simulink model "RLvali_2021bold"  (R2021b)
settings: Solver=ode15s  StartTime=0.0  StopTime=Tf  FixedStep=0.01  MaxStep=0.05  RelTol=0.5  AbsTol=0.5
model workspace (MATLAB code in the model file):
  | %---------------Critical values---------------%
  | angle_amp = pi/6; % Motor rotate amplitude, ref: pi/4
  | rotateCorrectionCoef = 1.158;
  | criticalFn = 2;
  | 
  | %------values for normalization---------------%
  | % values got by running manual gait
  | rotxNormGain = 1/0.1;
  | rotyNormGain = 1/0.05;
  | rotzNormGain = 1/0.1;
  | 
  | vxNormGain = 1/0.2;
  | vyNormGain = 1/0.2;
  | vzNormGain = 1/0.2;
  | 
  | FnNormGain = 1/15;
  | 
  | %--------values for check done---------------%
  | rotDone = pi/6; % 0.15;
  | legBendDone = pi/3; % actuator max bending angle
  | 
  | 
  | %---------------Robot parameters-------------%
  | % robot size
  | robot_width = 0.15;
  | robot_length = 0.22;
  | 
  | % floor parameters
  | floor_length = 2;
  | floor_width = 2;
  | 
  | % continuum actuator size
  | L_disk = 0.02944;% Disk side length (m)
  | R_w = L_disk/sqrt(3);
  | thickness_disk = 0.004; % Disk thickness (m)
  | thigh_length = 0.06;
  | R_core = 0.005; % Core radius (m)
  | length_core = 0.008; % Core length (m)
  | R_spool = 0.021; % 0.01944; % radius of the spool
  | spool_height = 0.022+0.015;
  | R_pulley = 1e-3;
  | spool_k = 0;
  | spool_d = 0;
  | hole_d = 4e-3;
  | 
  | % Material property
  | rho_PLA = 1.24e3;
  | rho = 1.19e3; % 1.19e3; % Density (kg/m^3)
  | % use rigid joints
  | Pz_stiff = 135000;
  | Pz_damping = 500;
  | S_stiff = 0.0239;
  | S_damping = 7.5e-5;
  | S_low_Bound = -20;
  | S_up_Bound = 20;
  | 
  | R_foot = 0.015; % foot radius (m)
  | 
  | % motor parameter
  | stall_T = 11.2/10; % 11.2 cm*kg, stall torque
  | t_60_deg = 0.2; % 0.09 s
  | V_nomrmal = 6; % corresponding normal voltage
  | Jr = 0.0001; %g*cm^2, robot inertia
  | 
  | % contact force
  | coef_static_friction = 0.315;
  | coef_dynamic_friction = 0.3;
  | crictic_velocity = 0.3; % m/s
  | contact_suf_stiff = 1000; % N/m
  | contact_suf_damp = 50; % N/(m/s)
  | contact_region_width = 2e-3; % m
  | spoolOpacity = 0;
  | tendonColor = [0.902 0.902 0.902];
  | tendonOpacity = 0.1;
  | 
  | % If use point masses
  | MMainFrame = 198; % g
  | MServoMotor = 50.55;
  | MMotorSupport = 12.1;
  | MSpool = 9.2;
  | 
  | % Robot total weight about 2 kg
  | MComposateLoad = 200;
  | 
  | MBuck = 40; % x2
  | MPCB_RPi = 141.3;
  | MLiBattery = 120; % x2
  | MPowerBank = 66.5;
  | isLoadVisible = 0.1;
  | 
  | 
  | MThigh = 26.7963;
  | MCore = 0.747699;
  | MDisk = 1.78642;
  | MFoot = 16.8232;
values from neighbouring files (symbols this model uses):
  N = ceil((A - 8) / (2.285 * abs(Wstop(1) - Wpass(1))))    [testit.m]
  Tf = 10    [longTest.m]    (also in singleTest.m)
  Ts = 0.05    [longTest.m]    (also in singleTest.m)
  x_norm_min = min(x,[],1)    [preprocessData.m]
  x_norm_range = max(x,[],1) - min(x,[],1)    [preprocessData.m]
  y_norm_min = min(y,[],1)    [preprocessData.m]
  y_norm_range = max(y,[],1) - min(y,[],1)    [preprocessData.m]
undefined symbols (not defined in the file or in its folder): alpha_b_gain, alpha_r_gain, DCMotor_K, EntropyList, EntropyWeightList, ExtParts, fnVariance, isCheckDone, isContactBoolean, isUseExtAct, MotorSupport, rotVariance, speedVariance, startAgentTime, TrackStarServo, VRef, WheelCAD, X, Y, Z, z_l_gain
libraries: sm_lib x311, nesl_utility x81, fl_lib x60, ee_lib x24, simulink x16, slpidlib x12, dspstat3 x2, rllib x1
(part 1 of 16)
settings Model: Creator=Qinglei Ji  LastModifiedBy=4DLab5
settings SolverCC: AutoScaleAbsTol=off  MaxConsecutiveZCs=100  MaxConsecutiveMinStep=10  DaesscMode=Fast  AutoInsertRateTranBlk=on
settings ExplorerConfigSet: InternalSimMechanicsExplorerSettings="<ExplorerConfiguration><canonicalview>default</canonicalview><AnimationSetting><BasePlaybackSpeed>1.0</BasePlaybackSpeed><PlaybackSpeedFactor>1.0</PlaybackSpeedFactor></AnimationSetting><TilePanel><TileInfo><Tiles Columns=\"1\" Count=\"1\" Rows=\"1\"><Column Weight=\"1\"/><Row Weight=\"1\"/><Tile Height=\"1\" Width=\"1\" X=\"0\" Y=\"0\"/></Tiles></TileInfo><SceneInfo><SceneViewer><BGColor><R>0.60000002384185791</R><G>0.60000002384185791</G><B>0.60000002384185791</B></BGColor><Camera><DoPerspective>off</DoPerspective><Position><X>-18.8331461547739707</X><Y>25.880517186070815</Y><Z>26.8100820833696147</Z></Position><Center><X>0.29785977478998571</X><Y>-0.293010908258582892</Y><Z>-0.346783787749327221</Z></Center><Up><X>0.517886432622382209</X><Y>-0.40389178028612327</Y><Z>0.754098848111419029</Z></Up><ViewLimDist>1</ViewLimDist><YLim>0.421333194645766129</YLim><XLim>0.456755011894746488</XLim></Camera></SceneViewer></SceneInfo></TilePanel><MechEditorPanel><Cameras/><GfxPanelCameraMap/><VideoCreator><PlaybackSpeedRatio>1.0</PlaybackSpeedRatio><FrameRate>60</FrameRate><VideoFormat>MPEG-4</VideoFormat><FrameSize>auto</FrameSize></VideoCreator></MechEditorPanel></ExplorerConfiguration>"

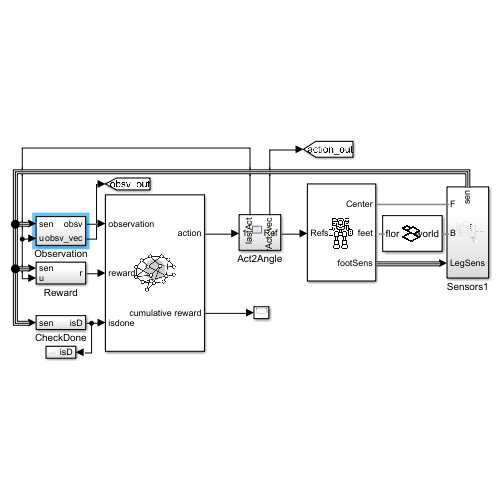
[thumbnail: Simulink's stored preview of the top-level diagram]
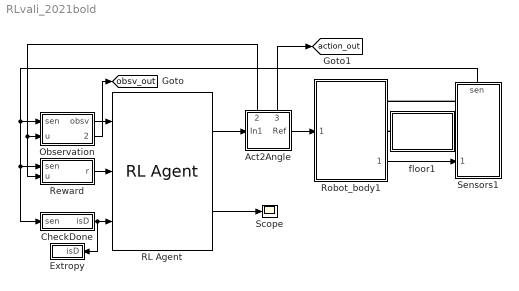
== system RLvali_2021bold ==
  Act2Angle : Subsystem
      settings: PortSchema="{\"entries\":[{\"content\":{\"sides\":[{\"content\":{\"connectorIds\":[\"In1\"]},\"type\":\"ConnectorPlacement.EquallySpacedRectSide\",\"uuid\":\"f23e08d3-9737-483d-bbfd-3ecb6f48fb39\"},{\"content\":{\"connectorIds\":[\"Out1\"],\"side\":\"RIGHT\"},\"type\":\"ConnectorPlacement.EquallySpacedRectSide\",\"uuid\":\"8d685ed7-5054-4615-a3e0-c1ab4f56a55e\"},{\"content\":{\"connectorIds\":[\"Out2\",\"Out3\"],\"side\":\"TOP\"},\"type\":\"ConnectorPlacement.EquallySpacedRectSide\",\"uuid\":\"34bb8f53-1c44-464f-ad5f-1618b85759f2\"}]},\"type\":\"ConnectorPlacement.EquallySpacedConnector\",\"uuid\":\"6728473f-c42e-49f1-b1f4-018a95208548\"}],\"packageUris\":[\"http://schema.mathworks.com/mf0/Connector/R2020b\"],\"version\":\"1.0\"}"
  CheckDone : Subsystem
  Extropy : Subsystem
  Observation : Subsystem
  RL Agent : rllib/RL Agent  Agent=agent  ExternalActionAsInput=off  ProvideCumRwd=on  TreatAsDirectFeedthrough=on
  Reward : Subsystem
  Robot_body1 : Subsystem
      settings: PortSchema="{\"entries\":[{\"content\":{\"sides\":[{\"content\":{\"connectorIds\":[]},\"type\":\"ConnectorPlacement.EquallySpacedRectSide\",\"uuid\":\"6da386a3-61dc-48ac-8951-5f405dad6f0b\"},{\"content\":{\"connectorIds\":[],\"side\":\"RIGHT\"},\"type\":\"ConnectorPlacement.EquallySpacedRectSide\",\"uuid\":\"f31d08fd-e336-4992-a7a1-a5f80310301f\"},{\"content\":{\"connectorIds\":[\"In1\"],\"side\":\"TOP\"},\"type\":\"ConnectorPlacement.EquallySpacedRectSide\",\"uuid\":\"e8d57c74-e878-4fd7-b952-570b3b82c07d\"},{\"content\":{\"connectorIds\":[\"RConn1\",\"RConn2\",\"Out1\"],\"side\":\"BOTTOM\"},\"type\":\"ConnectorPlacement.EquallySpacedRectSide\",\"uuid\":\"5cd044ae-e3eb-4740-b1cb-bb65851cb112\"}]},\"type\":\"ConnectorPlacement.EquallySpacedConnector\",\"uuid\":\"f9915cad-378a-4c2b-ad9c-362eed90ff8c\"}],\"packageUris\":[\"http://schema.mathworks.com/mf0/Connector/R2020b\"],\"version\":\"1.0\"}"
      mask Display: image('$imagefile'); % Use "Edit Image" on toolstrip to change.
  Scope : Scope
  Sensors1 : Subsystem
      settings: PortSchema="{\"entries\":[{\"content\":{\"sides\":[{\"content\":{\"connectorIds\":[\"LConn1\",\"LConn2\",\"In1\"]},\"type\":\"ConnectorPlacement.EquallySpacedRectSide\",\"uuid\":\"4b5ddd47-03f4-426a-88ee-d6acf531c637\"},{\"content\":{\"connectorIds\":[],\"side\":\"RIGHT\"},\"type\":\"ConnectorPlacement.EquallySpacedRectSide\",\"uuid\":\"f2192e31-fae6-4bce-a663-c668a18a2c9c\"},{\"content\":{\"connectorIds\":[\"Out1\"],\"side\":\"TOP\"},\"type\":\"ConnectorPlacement.EquallySpacedRectSide\",\"uuid\":\"20a91eaf-2ad2-4a0d-933a-434c603de7e7\"},{\"content\":{\"connectorIds\":[],\"side\":\"BOTTOM\"},\"type\":\"ConnectorPlacement.EquallySpacedRectSide\",\"uuid\":\"f2757d81-d7c7-43da-8561-08295a517c19\"}]},\"type\":\"ConnectorPlacement.EquallySpacedConnector\",\"uuid\":\"8ce371b8-5669-40c8-963e-855906aef91d\"}],\"packageUris\":[\"http://schema.mathworks.com/mf0/Connector/R2020b\"],\"version\":\"1.0\"}"
  floor1 : Subsystem
      mask Display: image('$imagefile'); % Use "Edit Image" on toolstrip to change.
  tag scope: action_out=global, obsv_out=global
  wires:
  Reward/1(r) -> RL Agent/2
  RL Agent/2 -> Scope/1
  Sensors1/1(sen) -> CheckDone/1(sen), Reward/1(sen), Observation/1(sen)
  CheckDone/1(isD) -> Extropy/1(isD), RL Agent/3
  Observation/1(obsv) -> RL Agent/1
  Act2Angle/1(Ref) -> Robot_body1/1(motorRefs)
  RL Agent/1 -> Act2Angle/1(In1)
  Observation/2(obsv_vec) -> [obsv_out]
  Act2Angle/3(currAct_vec) -> [action_out]
  Act2Angle/2(lastAct) -> Reward/2(u), Observation/2(u)
  Robot_body1/1(footSens) -> Sensors1/1(LegSens)
  connections:
  Sensors1/LConn1 -- Robot_body1/RConn1
  floor1/RConn1 -- Robot_body1/RConn2
  floor1/LConn1 -- Sensors1/LConn2

== system RLvali_2021bold/Act2Angle ==
  note: Learn motor ref
  In1 : Inport
  DecideToUseExt : Subsystem
  Delay : Delay  DelayLength=1  InitialCondition=[0.5;0.5;0.5;0.5]
  Human expert : Subsystem  Commented=on
  Human expert1 : Subsystem
  Subsystem1 : Subsystem  Commented=on
  Subsystem2 : Subsystem
  action2angle : Subsystem  Commented=on
  useExt? : Switch  Criteria=u2 > Threshold
  Ref : Outport
  lastAct : Outport  Port=2
  currAct_vec : Outport  Port=3
  wires:
  In1/1 -> useExt?/3  "Acts"
  Subsystem2/1(refs) -> Ref/1
  Delay/1 -> lastAct/1
  useExt?/1 -> Subsystem2/1(Acts), Delay/1, currAct_vec/1
  DecideToUseExt/1(Out1) -> useExt?/2
  Human expert1/1(Inport) -> useExt?/1

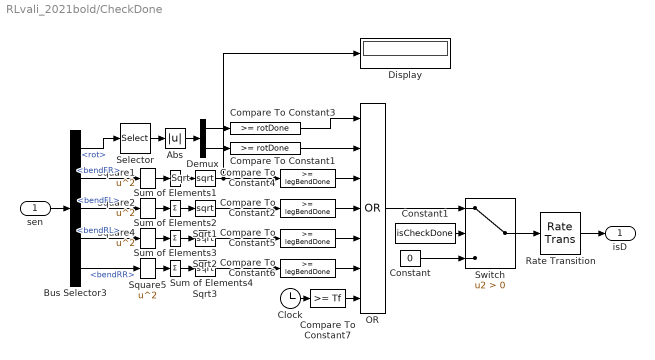
== system RLvali_2021bold/CheckDone ==
  sen : Inport
  Abs : Abs
  Bus Selector3 : BusSelector  OutputSignals=rot,SigsFromLegs.bendFR,SigsFromLegs.bendFL,SigsFromLegs.bendRL,SigsFromLegs.bendRR
  Clock : Clock
  Compare To Constant1 : simulink/Logic and Bit Operations/Compare To Constant  relop=>=  const=rotDone  OutDataTypeStr=boolean
  Compare To Constant{2,4..6} (4 alike) : simulink/Logic and Bit Operations/Compare To Constant  relop=>=  const=legBendDone  OutDataTypeStr=boolean
  Compare To Constant3 : simulink/Logic and Bit Operations/Compare To Constant  relop=>=  const=rotDone  OutDataTypeStr=boolean
  Compare To Constant7 : simulink/Logic and Bit Operations/Compare To Constant  relop=>=  const=Tf  OutDataTypeStr=boolean
  Constant : Constant  Value=0
  Constant1 : Constant  Value=isCheckDone
  Demux : Demux  Outputs=2
  Display : Display
  OR : Logic  Operator=OR  Inputs=7  AllPortsSameDT=off  OutDataTypeStr=boolean
  Rate Transition : RateTransition
  Selector : Selector  InputPortWidth=3  IndexOptions=Index vector (dialog)  Indices=[1 2]  OutputSizes=1
  Sqrt{,1..3} (4 alike) : Sqrt  SaturateOnIntegerOverflow=on
  Square{1..2,4..5} (4 alike) : Math  Operator=square  SignedPower=on  SaturateOnIntegerOverflow=on
  Sum of Elements{1..4} (4 alike) : Sum  Inputs=+
  Switch : Switch  Criteria=u2 > Threshold
  isD : Outport  VectorParamsAs1DForOutWhenUnconnected=off
  wires:
  Rate Transition/1 -> isD/1
  sen/1 -> Bus Selector3/1
  Bus Selector3/1 -> Selector/1  "<rot>"
  Compare To Constant3/1 -> OR/1
  Bus Selector3/2 -> Square1/1  "<bendFR>"
  Compare To Constant4/1 -> OR/3
  Square1/1 -> Sum of Elements1/1
  Sum of Elements1/1 -> Sqrt/1
  Sqrt/1 -> Compare To Constant4/1, Display/1
  Square2/1 -> Sum of Elements2/1
  Sqrt1/1 -> Compare To Constant2/1
  Sum of Elements2/1 -> Sqrt1/1
  Bus Selector3/3 -> Square2/1  "<bendFL>"
  Compare To Constant2/1 -> OR/4
  Square4/1 -> Sum of Elements3/1
  Sqrt2/1 -> Compare To Constant5/1
  Sum of Elements3/1 -> Sqrt2/1
  Bus Selector3/4 -> Square4/1  "<bendRL>"
  Compare To Constant5/1 -> OR/5
  Square5/1 -> Sum of Elements4/1
  Sqrt3/1 -> Compare To Constant6/1
  Sum of Elements4/1 -> Sqrt3/1
  Bus Selector3/5 -> Square5/1  "<bendRR>"
  Compare To Constant6/1 -> OR/6
  OR/1 -> Switch/1
  Switch/1 -> Rate Transition/1
  Constant/1 -> Switch/3
  Constant1/1 -> Switch/2
  Demux/1 -> Compare To Constant3/1
  Demux/2 -> Compare To Constant1/1
  Compare To Constant1/1 -> OR/2
  Clock/1 -> Compare To Constant7/1
  Compare To Constant7/1 -> OR/7
  Abs/1 -> Demux/1
  Selector/1 -> Abs/1

== system RLvali_2021bold/Extropy ==
  isD : Inport
  Clock : Clock
  Constant : Constant  Value=EntropyWeightList  SampleTime=Ts
  Constant2 : Constant  Value=EntropyList  SampleTime=Ts
  Display : Display
  MATLAB Function : MATLAB Function  TreatAsAtomicUnit=on  SystemSampleTime=Ts
  MATLAB Function1 : MATLAB Function  TreatAsAtomicUnit=on
  wires:
  Constant2/1 -> MATLAB Function/2(EntropyList)  "entropy"
  Constant/1 -> MATLAB Function/1(EntropyWeightList)  "entroWeight"
  isD/1 -> Display/1, MATLAB Function/3(isDone)
  [obsv_out] -> MATLAB Function1/2(obsv)
  [action_out] -> MATLAB Function1/3(act)
  Clock/1 -> MATLAB Function1/1(time)

== system RLvali_2021bold/Observation ==
  sen : Inport
  u : Inport  Port=2
  Mux : Mux
  Mux1 : Mux  Inputs=3
  Mux2 : Mux  Inputs=3
  Mux4 : Mux
  Rate Transition : RateTransition  OutPortSampleTime=Ts
  Subsystem : Subsystem
  contactConversion : Subsystem
  contactConversion1 : Subsystem
  contactConversion2 : Subsystem
  contactConversion3 : Subsystem
  correct : Subsystem  Commented=on
  rotNoise : Subsystem
  rotNoise1 : Subsystem
  rotNoise2 : Subsystem
  speednoise : Subsystem
  speednoise1 : Subsystem
  speednoise2 : Subsystem
  obsv : Outport  VectorParamsAs1DForOutWhenUnconnected=off
  obsv_vec : Outport  Port=2  VectorParamsAs1DForOutWhenUnconnected=off
  wires:
  Mux/1 -> Rate Transition/1
  Rate Transition/1 -> obsv/1
  u/1 -> Mux/4
  Mux1/1 -> Mux/1
  Mux2/1 -> Mux/2
  contactConversion/1(FnOut) -> Mux4/1
  contactConversion1/1(FnOut) -> Mux4/2
  contactConversion2/1(FnOut) -> Mux4/3
  contactConversion3/1(FnOut) -> Mux4/4
  Mux4/1 -> Mux/3
  speednoise/1(Out1) -> Mux2/1
  speednoise1/1(Out1) -> Mux2/2
  speednoise2/1(Out1) -> Mux2/3
  rotNoise/1(Out1) -> Mux1/1
  rotNoise1/1(Out1) -> Mux1/2
  rotNoise2/1(Out1) -> Mux1/3
  sen/1 -> Subsystem/1(In1)
  Subsystem/1(obsv_vec) -> obsv_vec/1
  Subsystem/2(norm) -> rotNoise/1(<vx>)
  Subsystem/3(norm1) -> rotNoise1/1(<vx>)
  Subsystem/4(norm2) -> rotNoise2/1(<vx>)
  Subsystem/5(norm3) -> speednoise/1(<vx>)
  Subsystem/6(norm4) -> speednoise1/1(<vx>)
  Subsystem/7(norm5) -> speednoise2/1(<vx>)
  Subsystem/8(norm6) -> contactConversion/1(Fn)
  Subsystem/9(norm7) -> contactConversion1/1(Fn)
  Subsystem/10(norm8) -> contactConversion2/1(Fn)
  Subsystem/11(norm9) -> contactConversion3/1(Fn)

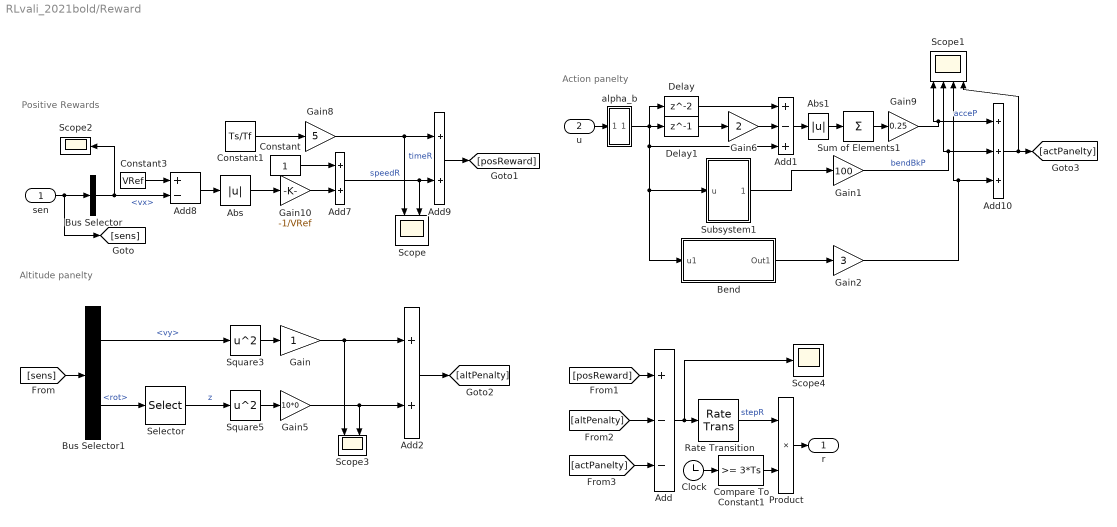
== system RLvali_2021bold/Reward ==
  note: Action panelty
  note: Altitude panelty
  note: Positive Rewards
  sen : Inport
  u : Inport  Port=2
  Abs : Abs
  Abs1 : Abs
  Add : Sum  Inputs=+--
  Add1 : Sum  Inputs=+-+
  Add10 : Sum  Inputs=+++
  Add2 : Sum
  Add7 : Sum
  Add8 : Sum  Inputs=+-
  Add9 : Sum
  Bend : Subsystem
  Bus Selector : BusSelector  OutputSignals=vx
  Bus Selector1 : BusSelector  OutputSignals=vy,rot
  Clock : Clock
  Compare To Constant1 : simulink/Logic and Bit Operations/Compare To Constant  relop=>=  const=3*Ts  OutDataTypeStr=boolean
  Constant : Constant
  Constant1 : Constant  Value=Ts/Tf
  Constant3 : Constant  Value=VRef
  Delay : Delay  InitialCondition=0.5
  Delay1 : Delay  DelayLength=1  InitialCondition=0.5
  Gain : Gain
  Gain1 : Gain  Gain=100
  Gain10 : Gain  Gain=-1/VRef
  Gain2 : Gain  Gain=3
  Gain5 : Gain  Gain=10*0
  Gain6 : Gain  Gain=2
  Gain8 : Gain  Gain=5
  Gain9 : Gain  Gain=0.25
  Product : Product
  Rate Transition : RateTransition  OutPortSampleTime=Ts
  Scope : Scope  NumInputPorts=2
  Scope1 : Scope  NumInputPorts=4
  Scope2 : Scope
  Scope3 : Scope  NumInputPorts=2
  Scope4 : Scope
  Selector : Selector  InputPortWidth=3  IndexOptions=Index vector (dialog)  Indices=[3]  OutputSizes=1
  Square3 : Math  Operator=square  SignedPower=on  SaturateOnIntegerOverflow=on
  Square5 : Math  Operator=square  SignedPower=on  SaturateOnIntegerOverflow=on
  Subsystem1 : Subsystem
  Sum of Elements1 : Sum  Inputs=+
  alpha_b : Subsystem
  r : Outport  VectorParamsAs1DForOutWhenUnconnected=off
  wires:
  sen/1 -> Bus Selector/1, [sens]
  Square3/1 -> Gain/1
  Square5/1 -> Gain5/1
  Selector/1 -> Square5/1  "z"
  Gain/1 -> Scope3/1, Add2/1
  Add/1 -> Scope4/1, Rate Transition/1
  Constant1/1 -> Gain8/1
  Delay/1 -> Add1/1
  Gain6/1 -> Add1/2
  Add1/1 -> Abs1/1
  Abs1/1 -> Sum of Elements1/1
  Delay1/1 -> Gain6/1
  Sum of Elements1/1 -> Gain9/1
  Clock/1 -> Compare To Constant1/1
  Compare To Constant1/1 -> Product/2
  Rate Transition/1 -> Product/1  "stepR"
  Product/1 -> r/1
  [sens] -> Bus Selector1/1
  Gain8/1 -> Add9/1, Scope/1  "timeR"
  Add9/1 -> [posReward]
  Bus Selector1/1 -> Square3/1  "<vy>"
  Bus Selector1/2 -> Selector/1  "<rot>"
  Gain5/1 -> Add2/2, Scope3/2
  Add2/1 -> [altPenalty]
  Gain9/1 -> Add10/1, Scope1/1  "acceP"
  [posReward] -> Add/1
  [altPenalty] -> Add/2
  [actPanelty] -> Add/3
  Add8/1 -> Abs/1
  Constant3/1 -> Add8/1
  Add7/1 -> Scope/2, Add9/2  "speedR"
  Gain10/1 -> Add7/2
  Abs/1 -> Gain10/1
  Constant/1 -> Add7/1
  Subsystem1/1(Out1) -> Gain1/1
  Gain1/1 -> Add10/2, Scope1/2  "bendBkP"
  Add10/1 -> Scope1/4, [actPanelty]
  alpha_b/1(b) -> Bend/1(u1), Subsystem1/1(u), Add1/3, Delay/1, Delay1/1
  u/1 -> alpha_b/1(u)
  Bend/1(Out1) -> Gain2/1
  Gain2/1 -> Scope1/3, Add10/3
  Bus Selector/1 -> Scope2/1, Add8/2  "<vx>"

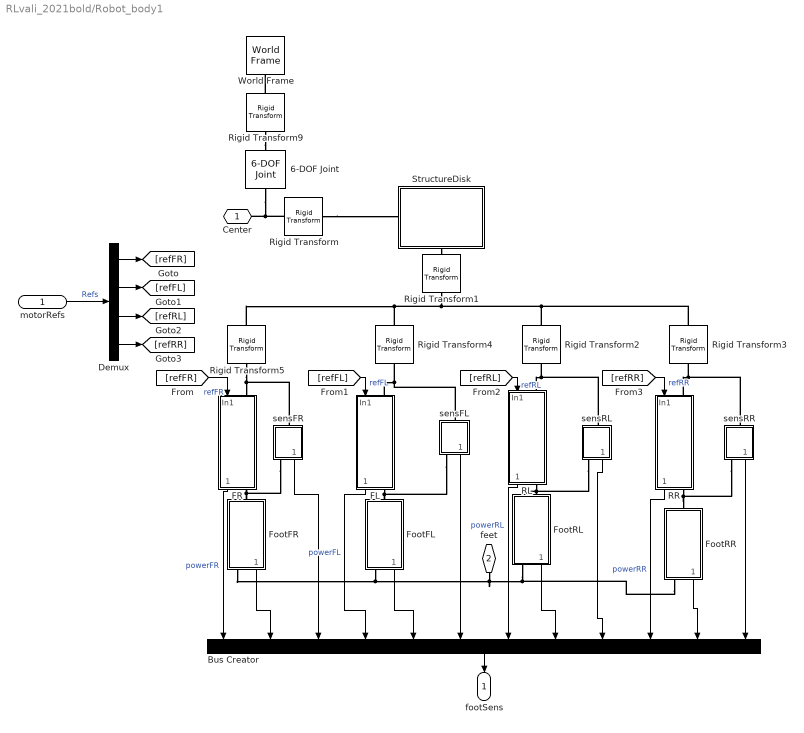
== system RLvali_2021bold/Robot_body1 ==
  motorRefs : Inport
  6-DOF Joint : sm_lib/Joints/6-DOF Joint  JointMode=Normal  SenseConstraintForce=off  SenseConstraintForceX=off  SenseConstraintForceY=off  SenseConstraintForceZ=off  SenseConstraintTorque=off  SenseConstraintTorqueX=off  SenseConstraintTorqueY=off  SenseConstraintTorqueZ=off  SenseTotalForce=off  SenseTotalForceX=off  SenseTotalForceY=off  SenseTotalForceZ=off  SenseTotalTorque=off  SenseTotalTorqueX=off  SenseTotalTorqueY=off  SenseTotalTorqueZ=off  CompositeWrenchDir=FollowerOnBase  CompositeWrenchFrame=BaseFrame  PxEquilibriumPosition=0  PxEquilibriumPositionUnits=m  PxSpringStiffness=0  PxSpringStiffnessUnits=N/m  PxDampingCoefficient=0  PxDampingCoefficientUnits=N/(m/s)  PxTorqueActuationMode=NoTorque  PxMotionActuationMode=ComputedMotion  PxSensePosition=off  PxSenseVelocity=off  PxSenseAcceleration=off  PxSenseTorqueForce=off  PxSenseLowerLimitTorqueForce=off  PxSenseUpperLimitTorqueForce=off  PxLowerLimitSpecify=off  PxLowerLimitBound=-1  PxLowerLimitBoundUnits=m  PxLowerLimitStiffness=1e6  PxLowerLimitStiffnessUnits=N/m  PxLowerLimitDamping=1e3  PxLowerLimitDampingUnits=N/(m/s)  PxLowerLimitTransitionRegionWidth=1e-4  PxLowerLimitTransitionRegionWidthUnits=m  PxUpperLimitSpecify=off  PxUpperLimitBound=1  PxUpperLimitBoundUnits=m  PxUpperLimitStiffness=1e6  PxUpperLimitStiffnessUnits=N/m  PxUpperLimitDamping=1e3  PxUpperLimitDampingUnits=N/(m/s)  PxUpperLimitTransitionRegionWidth=1e-4  PxUpperLimitTransitionRegionWidthUnits=m  PxPositionTargetSpecify=off  PxPositionTargetPriority=High  PxPositionTargetValue=0  PxPositionTargetValueUnits=m  PxVelocityTargetSpecify=off  PxVelocityTargetPriority=High  PxVelocityTargetValue=0  PxVelocityTargetValueUnits=m/s  PyEquilibriumPosition=0  PyEquilibriumPositionUnits=m  PySpringStiffness=0  PySpringStiffnessUnits=N/m  PyDampingCoefficient=0  PyDampingCoefficientUnits=N/(m/s)  PyTorqueActuationMode=NoTorque  PyMotionActuationMode=ComputedMotion  PySensePosition=off  PySenseVelocity=off  PySenseAcceleration=off  PySenseTorqueForce=off  PySenseLowerLimitTorqueForce=off  PySenseUpperLimitTorqueForce=off  PyLowerLimitSpecify=off  PyLowerLimitBound=-1  PyLowerLimitBoundUnits=m  PyLowerLimitStiffness=1e6  PyLowerLimitStiffnessUnits=N/m  PyLowerLimitDamping=1e3  PyLowerLimitDampingUnits=N/(m/s)  PyLowerLimitTransitionRegionWidth=1e-4  PyLowerLimitTransitionRegionWidthUnits=m  PyUpperLimitSpecify=off  PyUpperLimitBound=1  PyUpperLimitBoundUnits=m  PyUpperLimitStiffness=1e6  PyUpperLimitStiffnessUnits=N/m  PyUpperLimitDamping=1e3  PyUpperLimitDampingUnits=N/(m/s)  PyUpperLimitTransitionRegionWidth=1e-4  PyUpperLimitTransitionRegionWidthUnits=m  PyPositionTargetSpecify=off  PyPositionTargetPriority=High  PyPositionTargetValue=0  PyPositionTargetValueUnits=m  PyVelocityTargetSpecify=off  PyVelocityTargetPriority=High  PyVelocityTargetValue=0  PyVelocityTargetValueUnits=m/s  PzEquilibriumPosition=0  PzEquilibriumPositionUnits=m  PzSpringStiffness=0  PzSpringStiffnessUnits=N/m  PzDampingCoefficient=0  PzDampingCoefficientUnits=N/(m/s)  PzTorqueActuationMode=NoTorque  PzMotionActuationMode=ComputedMotion  PzSensePosition=off  PzSenseVelocity=off  PzSenseAcceleration=off  PzSenseTorqueForce=off  PzSenseLowerLimitTorqueForce=off  PzSenseUpperLimitTorqueForce=off  PzLowerLimitSpecify=off  PzLowerLimitBound=-1  PzLowerLimitBoundUnits=m  PzLowerLimitStiffness=1e6  PzLowerLimitStiffnessUnits=N/m  PzLowerLimitDamping=1e3  PzLowerLimitDampingUnits=N/(m/s)  PzLowerLimitTransitionRegionWidth=1e-4  PzLowerLimitTransitionRegionWidthUnits=m  PzUpperLimitSpecify=off  PzUpperLimitBound=1  PzUpperLimitBoundUnits=m  PzUpperLimitStiffness=1e6  PzUpperLimitStiffnessUnits=N/m  PzUpperLimitDamping=1e3  PzUpperLimitDampingUnits=N/(m/s)  PzUpperLimitTransitionRegionWidth=1e-4  PzUpperLimitTransitionRegionWidthUnits=m  PzPositionTargetSpecify=off  PzPositionTargetPriority=High  PzPositionTargetValue=0  PzPositionTargetValueUnits=m  PzVelocityTargetSpecify=off  PzVelocityTargetPriority=High  PzVelocityTargetValue=0  PzVelocityTargetValueUnits=m/s  SphDefPosRotationMethod=None  SphDefPosRotationAngleUnits=deg  SphDefPosRotationStandardAxis=+Z  SphDefPosRotationAngle=0.0  SphDefPosRotationArbitraryAxis=[0 0 1]  SphDefPosFollAlignAxisA=+X  SphDefPosBaseAlignAxisA=+Y  SphDefPosFollAlignAxisB=+Y  SphDefPosBaseAlignAxisB=+Z  SphDefPosRotationSequenceAxes=FollowerAxes  SphDefPosRotationSequence=XYX  SphDefPosRotationSequenceAngles=[0 0 0]  SphDefPosRotationSequenceAnglesUnits=deg  SphDefPosRotationMatrix=[1 0 0; 0 1 0; 0 0 1]  SphEqPosRotationMethod=None  SphEqPosRotationAngleUnits=deg  SphEqPosRotationStandardAxis=+Z  SphEqPosRotationAngle=0.0  SphEqPosRotationArbitraryAxis=[0 0 1]  SphEqPosFollAlignAxisA=+X  SphEqPosBaseAlignAxisA=+Y  SphEqPosFollAlignAxisB=+Y  SphEqPosBaseAlignAxisB=+Z  SphEqPosRotationSequenceAxes=FollowerAxes  SphEqPosRotationSequence=XYX  SphEqPosRotationSequenceAngles=[0 0 0]  SphEqPosRotationSequenceAnglesUnits=deg  SphEqPosRotationMatrix=[1 0 0; 0 1 0; 0 0 1]  SphSpringStiffness=0  SphSpringStiffnessUnits=N*m/deg  SphDampingCoefficient=0  SphDampingCoefficientUnits=N*m/(deg/s)  SphActuateTorqueX=off  SphActuateTorqueY=off  SphActuateTorqueZ=off  SphActuateTorque=off  SphTorqueActuationMode=NoTorque  SphMotionActuationMode=ComputedMotion  SphActuationFrame=BaseFrame  SphSensePosition=off  SphSenseVelocityX=off  SphSenseVelocityY=off  SphSenseVelocityZ=off  SphSenseVelocity=off  SphSenseAccelerationX=off  SphSenseAccelerationY=off  SphSenseAccelerationZ=off  SphSenseAcceleration=off  SphSenseTorqueX=off  SphSenseTorqueY=off  SphSenseTorqueZ=off  SphSenseTorqueForce=off  SphSenseLowerLimitTorqueMag=off  SphSenseUpperLimitTorqueMag=off  SphSensingFrame=BaseFrame  SphLowerLimitSpecify=off  SphLowerLimitBound=15  SphLowerLimitBoundUnits=deg  SphLowerLimitStiffness=1e4  SphLowerLimitStiffnessUnits=N*m/deg  SphLowerLimitDamping=10  SphLowerLimitDampingUnits=N*m/(deg/s)  SphLowerLimitTransitionRegionWidth=0.1  SphLowerLimitTransitionRegionWidthUnits=deg  SphUpperLimitSpecify=off  SphUpperLimitBound=45  SphUpperLimitBoundUnits=deg  SphUpperLimitStiffness=1e4  SphUpperLimitStiffnessUnits=N*m/deg  SphUpperLimitDamping=10  SphUpperLimitDampingUnits=N*m/(deg/s)  SphUpperLimitTransitionRegionWidth=0.1  SphUpperLimitTransitionRegionWidthUnits=deg  SphPositionTargetRotationMethod=None  SphPositionTargetRotationAngleUnits=deg  SphPositionTargetRotationStandardAxis=+Z  SphPositionTargetRotationAngle=0.0  SphPositionTargetRotationArbitraryAxis=[0 0 1]  SphPositionTargetFollAlignAxisA=+X  SphPositionTargetBaseAlignAxisA=+Y  SphPositionTargetFollAlignAxisB=+Y  SphPositionTargetBaseAlignAxisB=+Z  SphPositionTargetRotationSequenceAxes=FollowerAxes  SphPositionTargetRotationSequence=XYX  SphPositionTargetRotationSequenceAngles=[0 0 0]  SphPositionTargetRotationSequenceAnglesUnits=deg  SphPositionTargetRotationMatrix=[1 0 0; 0 1 0; 0 0 1]  SphPositionTargetSpecify=off  SphPositionTargetPriority=High  SphVelocityTargetValue=[0 0 0]  SphVelocityTargetValueUnits=deg/s  SphVelocityTargetSpecify=off  SphVelocityTargetPriority=High  SphVelocityTargetInFollowerFrame=on
  Bus Creator : BusCreator  Inputs=12
  Demux : Demux
  FL : Subsystem
  FR : Subsystem
  FootFL : Subsystem
      settings: PortSchema="{\"entries\":[{\"content\":{\"sides\":[{\"content\":{\"connectorIds\":[\"LConn1\",\"Out1\"]},\"type\":\"ConnectorPlacement.EquallySpacedRectSide\",\"uuid\":\"0bb1f20c-4b5e-487a-8abf-3e1f2fef015b\"},{\"content\":{\"connectorIds\":[\"RConn1\"],\"side\":\"RIGHT\"},\"type\":\"ConnectorPlacement.EquallySpacedRectSide\",\"uuid\":\"5d13e6ab-8a90-4d8e-960d-d3cf2c1ae97d\"},{\"content\":{\"connectorIds\":[],\"side\":\"TOP\"},\"type\":\"ConnectorPlacement.EquallySpacedRectSide\",\"uuid\":\"95bd9573-7fea-4bcb-a448-c8ab92610e8b\"},{\"content\":{\"connectorIds\":[],\"side\":\"BOTTOM\"},\"type\":\"ConnectorPlacement.EquallySpacedRectSide\",\"uuid\":\"976c40b0-0fd4-4a26-8e09-25e540e36d50\"}]},\"type\":\"ConnectorPlacement.EquallySpacedConnector\",\"uuid\":\"5d9c26bf-393c-4096-afaf-0ed92cf9ce69\"}],\"packageUris\":[\"http://schema.mathworks.com/mf0/Connector/R2020b\"],\"version\":\"1.0\"}"
  FootFR : Subsystem
      settings: PortSchema="{\"entries\":[{\"content\":{\"sides\":[{\"content\":{\"connectorIds\":[\"LConn1\",\"Out1\"]},\"type\":\"ConnectorPlacement.EquallySpacedRectSide\",\"uuid\":\"0bb1f20c-4b5e-487a-8abf-3e1f2fef015b\"},{\"content\":{\"connectorIds\":[\"RConn1\"],\"side\":\"RIGHT\"},\"type\":\"ConnectorPlacement.EquallySpacedRectSide\",\"uuid\":\"5d13e6ab-8a90-4d8e-960d-d3cf2c1ae97d\"},{\"content\":{\"connectorIds\":[],\"side\":\"TOP\"},\"type\":\"ConnectorPlacement.EquallySpacedRectSide\",\"uuid\":\"95bd9573-7fea-4bcb-a448-c8ab92610e8b\"},{\"content\":{\"connectorIds\":[],\"side\":\"BOTTOM\"},\"type\":\"ConnectorPlacement.EquallySpacedRectSide\",\"uuid\":\"976c40b0-0fd4-4a26-8e09-25e540e36d50\"}]},\"type\":\"ConnectorPlacement.EquallySpacedConnector\",\"uuid\":\"5d9c26bf-393c-4096-afaf-0ed92cf9ce69\"}],\"packageUris\":[\"http://schema.mathworks.com/mf0/Connector/R2020b\"],\"version\":\"1.0\"}"
  FootRL : Subsystem
      settings: PortSchema="{\"entries\":[{\"content\":{\"sides\":[{\"content\":{\"connectorIds\":[\"LConn1\",\"Out1\"]},\"type\":\"ConnectorPlacement.EquallySpacedRectSide\",\"uuid\":\"0bb1f20c-4b5e-487a-8abf-3e1f2fef015b\"},{\"content\":{\"connectorIds\":[\"RConn1\"],\"side\":\"RIGHT\"},\"type\":\"ConnectorPlacement.EquallySpacedRectSide\",\"uuid\":\"5d13e6ab-8a90-4d8e-960d-d3cf2c1ae97d\"},{\"content\":{\"connectorIds\":[],\"side\":\"TOP\"},\"type\":\"ConnectorPlacement.EquallySpacedRectSide\",\"uuid\":\"95bd9573-7fea-4bcb-a448-c8ab92610e8b\"},{\"content\":{\"connectorIds\":[],\"side\":\"BOTTOM\"},\"type\":\"ConnectorPlacement.EquallySpacedRectSide\",\"uuid\":\"976c40b0-0fd4-4a26-8e09-25e540e36d50\"}]},\"type\":\"ConnectorPlacement.EquallySpacedConnector\",\"uuid\":\"5d9c26bf-393c-4096-afaf-0ed92cf9ce69\"}],\"packageUris\":[\"http://schema.mathworks.com/mf0/Connector/R2020b\"],\"version\":\"1.0\"}"
  FootRR : Subsystem
      settings: PortSchema="{\"entries\":[{\"content\":{\"sides\":[{\"content\":{\"connectorIds\":[\"LConn1\",\"Out1\"]},\"type\":\"ConnectorPlacement.EquallySpacedRectSide\",\"uuid\":\"0bb1f20c-4b5e-487a-8abf-3e1f2fef015b\"},{\"content\":{\"connectorIds\":[\"RConn1\"],\"side\":\"RIGHT\"},\"type\":\"ConnectorPlacement.EquallySpacedRectSide\",\"uuid\":\"5d13e6ab-8a90-4d8e-960d-d3cf2c1ae97d\"},{\"content\":{\"connectorIds\":[],\"side\":\"TOP\"},\"type\":\"ConnectorPlacement.EquallySpacedRectSide\",\"uuid\":\"95bd9573-7fea-4bcb-a448-c8ab92610e8b\"},{\"content\":{\"connectorIds\":[],\"side\":\"BOTTOM\"},\"type\":\"ConnectorPlacement.EquallySpacedRectSide\",\"uuid\":\"976c40b0-0fd4-4a26-8e09-25e540e36d50\"}]},\"type\":\"ConnectorPlacement.EquallySpacedConnector\",\"uuid\":\"5d9c26bf-393c-4096-afaf-0ed92cf9ce69\"}],\"packageUris\":[\"http://schema.mathworks.com/mf0/Connector/R2020b\"],\"version\":\"1.0\"}"
  RL : Subsystem
  RR : Subsystem
  Rigid Transform : sm_lib/Frames and Transforms/Rigid Transform  TranslationMethod=None  TranslationStandardOffset=0.1  TranslationLengthUnit=m  TranslationStandardAxis=+Z  TranslationCartesianOffset=[0 0 0]  TranslationROffset=0  TranslationROffsetUnits=m  TranslationZOffset=0  TranslationZOffsetUnits=m  TranslationThetaOffset=0  TranslationThetaOffsetUnits=deg  RotationMethod=StandardAxis  RotationAngleUnits=deg  RotationStandardAxis=-Z  RotationAngle=90  RotationArbitraryAxis=[0 0 1]  FollAlignAxisA=+X  BaseAlignAxisA=+Z  FollAlignAxisB=+Y  BaseAlignAxisB=+Z  RotationSequenceAxes=FollowerAxes  RotationSequence=XYX  RotationSequenceAngles=[0 0 0]  RotationSequenceAnglesUnits=deg  RotationMatrix=[1 0 0; 0 1 0; 0 0 1]
  Rigid Transform1 : sm_lib/Frames and Transforms/Rigid Transform  TranslationMethod=None  TranslationStandardOffset=0.1  TranslationLengthUnit=m  TranslationStandardAxis=+Z  TranslationCartesianOffset=[0 0 0]  TranslationROffset=0  TranslationROffsetUnits=m  TranslationZOffset=0  TranslationZOffsetUnits=m  TranslationThetaOffset=0  TranslationThetaOffsetUnits=deg  RotationMethod=StandardAxis  RotationAngleUnits=deg  RotationStandardAxis=+Z  RotationAngle=90  RotationArbitraryAxis=[0 0 1]  FollAlignAxisA=+X  BaseAlignAxisA=+Z  FollAlignAxisB=+Y  BaseAlignAxisB=+Z  RotationSequenceAxes=FollowerAxes  RotationSequence=XYX  RotationSequenceAngles=[0 0 0]  RotationSequenceAnglesUnits=deg  RotationMatrix=[1 0 0; 0 1 0; 0 0 1]
  Rigid Transform2 : sm_lib/Frames and Transforms/Rigid Transform  TranslationMethod=Cartesian  TranslationStandardOffset=0  TranslationLengthUnit=m  TranslationStandardAxis=+Z  TranslationCartesianOffset=[robot_length/2 -robot_width/2 0]  TranslationROffset=0  TranslationROffsetUnits=m  TranslationZOffset=0  TranslationZOffsetUnits=m  TranslationThetaOffset=0  TranslationThetaOffsetUnits=deg  RotationMethod=None  RotationAngleUnits=deg  RotationStandardAxis=+Z  RotationAngle=0.0  RotationArbitraryAxis=[0 0 1]  FollAlignAxisA=+X  BaseAlignAxisA=+Y  FollAlignAxisB=+Y  BaseAlignAxisB=+Z  RotationSequenceAxes=FollowerAxes  RotationSequence=XYX  RotationSequenceAngles=[0 0 0]  RotationSequenceAnglesUnits=deg  RotationMatrix=[1 0 0; 0 1 0; 0 0 1]
  Rigid Transform3 : sm_lib/Frames and Transforms/Rigid Transform  TranslationMethod=Cartesian  TranslationStandardOffset=0  TranslationLengthUnit=m  TranslationStandardAxis=+Z  TranslationCartesianOffset=[robot_length/2 robot_width/2 0]  TranslationROffset=0  TranslationROffsetUnits=m  TranslationZOffset=0  TranslationZOffsetUnits=m  TranslationThetaOffset=0  TranslationThetaOffsetUnits=deg  RotationMethod=None  RotationAngleUnits=deg  RotationStandardAxis=+Z  RotationAngle=0.0  RotationArbitraryAxis=[0 0 1]  FollAlignAxisA=+X  BaseAlignAxisA=+Y  FollAlignAxisB=+Y  BaseAlignAxisB=+Z  RotationSequenceAxes=FollowerAxes  RotationSequence=XYX  RotationSequenceAngles=[0 0 0]  RotationSequenceAnglesUnits=deg  RotationMatrix=[1 0 0; 0 1 0; 0 0 1]
  Rigid Transform4 : sm_lib/Frames and Transforms/Rigid Transform  TranslationMethod=Cartesian  TranslationStandardOffset=0  TranslationLengthUnit=m  TranslationStandardAxis=+Z  TranslationCartesianOffset=[-robot_length/2 -robot_width/2 0]  TranslationROffset=0  TranslationROffsetUnits=m  TranslationZOffset=0  TranslationZOffsetUnits=m  TranslationThetaOffset=0  TranslationThetaOffsetUnits=deg  RotationMethod=None  RotationAngleUnits=deg  RotationStandardAxis=+Z  RotationAngle=0.0  RotationArbitraryAxis=[0 0 1]  FollAlignAxisA=+X  BaseAlignAxisA=+Y  FollAlignAxisB=+Y  BaseAlignAxisB=+Z  RotationSequenceAxes=FollowerAxes  RotationSequence=XYX  RotationSequenceAngles=[0 0 0]  RotationSequenceAnglesUnits=deg  RotationMatrix=[1 0 0; 0 1 0; 0 0 1]
  Rigid Transform5 : sm_lib/Frames and Transforms/Rigid Transform  TranslationMethod=Cartesian  TranslationStandardOffset=0  TranslationLengthUnit=m  TranslationStandardAxis=+Z  TranslationCartesianOffset=[-robot_length/2 robot_width/2 0]  TranslationROffset=0  TranslationROffsetUnits=m  TranslationZOffset=0  TranslationZOffsetUnits=m  TranslationThetaOffset=0  TranslationThetaOffsetUnits=deg  RotationMethod=None  RotationAngleUnits=deg  RotationStandardAxis=+Z  RotationAngle=0.0  RotationArbitraryAxis=[0 0 1]  FollAlignAxisA=+X  BaseAlignAxisA=+Y  FollAlignAxisB=+Y  BaseAlignAxisB=+Z  RotationSequenceAxes=FollowerAxes  RotationSequence=XYX  RotationSequenceAngles=[0 0 0]  RotationSequenceAnglesUnits=deg  RotationMatrix=[1 0 0; 0 1 0; 0 0 1]
  Rigid Transform9 : sm_lib/Frames and Transforms/Rigid Transform  TranslationMethod=Cartesian  TranslationStandardOffset=0  TranslationLengthUnit=m  TranslationStandardAxis=+Z  TranslationCartesianOffset=[0 0 0.155]  TranslationROffset=0  TranslationROffsetUnits=m  TranslationZOffset=0  TranslationZOffsetUnits=m  TranslationThetaOffset=0  TranslationThetaOffsetUnits=deg  RotationMethod=StandardAxis  RotationAngleUnits=deg  RotationStandardAxis=+Y  RotationAngle=0  RotationArbitraryAxis=[0 0 1]  FollAlignAxisA=+X  BaseAlignAxisA=+Y  FollAlignAxisB=+Y  BaseAlignAxisB=+Z  RotationSequenceAxes=FollowerAxes  RotationSequence=XYX  RotationSequenceAngles=[0 0 0]  RotationSequenceAnglesUnits=deg  RotationMatrix=[1 0 0; 0 1 0; 0 0 1]
  StructureDisk : Subsystem
      settings: PortSchema="{\"entries\":[{\"content\":{\"sides\":[{\"content\":{\"connectorIds\":[]},\"type\":\"ConnectorPlacement.EquallySpacedRectSide\",\"uuid\":\"983b4593-33f8-4f05-8496-f6a680e0506a\"},{\"content\":{\"connectorIds\":[\"RConn1\"],\"side\":\"RIGHT\"},\"type\":\"ConnectorPlacement.EquallySpacedRectSide\",\"uuid\":\"dd1cb835-99ed-40eb-9457-9a76e9b19610\"},{\"content\":{\"connectorIds\":[\"LConn1\"],\"side\":\"TOP\"},\"type\":\"ConnectorPlacement.EquallySpacedRectSide\",\"uuid\":\"c15c4885-45e6-4882-9e3a-df9802ff439f\"}]},\"type\":\"ConnectorPlacement.EquallySpacedConnector\",\"uuid\":\"19826241-0a68-4e2d-83d2-fcb027292ea7\"}],\"packageUris\":[\"http://schema.mathworks.com/mf0/Connector/R2020b\"],\"version\":\"1.0\"}"
      mask DialogControl DescTextVar Prompt: StructureDisk.png
      mask Display: image('$imagefile'); % Use "Edit Image" on toolstrip to change.
  World Frame : sm_lib/Frames and Transforms/World Frame
  sensFL : Subsystem
      settings: PortSchema="{\"entries\":[{\"content\":{\"sides\":[{\"content\":{\"connectorIds\":[]},\"type\":\"ConnectorPlacement.EquallySpacedRectSide\",\"uuid\":\"bd83465d-2bef-45ec-b31a-ccd96dc04922\"},{\"content\":{\"connectorIds\":[],\"side\":\"RIGHT\"},\"type\":\"ConnectorPlacement.EquallySpacedRectSide\",\"uuid\":\"7d39c37e-7359-45a9-8850-f640f6442332\"},{\"content\":{\"connectorIds\":[\"LConn1\"],\"side\":\"TOP\"},\"type\":\"ConnectorPlacement.EquallySpacedRectSide\",\"uuid\":\"9171d6ae-b8cc-4ed2-b32d-fb0addba6640\"},{\"content\":{\"connectorIds\":[\"Out1\",\"RConn1\"],\"side\":\"BOTTOM\"},\"type\":\"ConnectorPlacement.EquallySpacedRectSide\",\"uuid\":\"6d61618f-1cbe-4c91-8d9a-cf1c63ddd154\"}]},\"type\":\"ConnectorPlacement.EquallySpacedConnector\",\"uuid\":\"3aecd3e6-ec94-4a95-ad20-92352af1806b\"}],\"packageUris\":[\"http://schema.mathworks.com/mf0/Connector/R2020b\"],\"version\":\"1.0\"}"
  sensFR : Subsystem
      settings: PortSchema="{\"entries\":[{\"content\":{\"sides\":[{\"content\":{\"connectorIds\":[]},\"type\":\"ConnectorPlacement.EquallySpacedRectSide\",\"uuid\":\"bd83465d-2bef-45ec-b31a-ccd96dc04922\"},{\"content\":{\"connectorIds\":[],\"side\":\"RIGHT\"},\"type\":\"ConnectorPlacement.EquallySpacedRectSide\",\"uuid\":\"7d39c37e-7359-45a9-8850-f640f6442332\"},{\"content\":{\"connectorIds\":[\"LConn1\"],\"side\":\"TOP\"},\"type\":\"ConnectorPlacement.EquallySpacedRectSide\",\"uuid\":\"9171d6ae-b8cc-4ed2-b32d-fb0addba6640\"},{\"content\":{\"connectorIds\":[\"Out1\",\"RConn1\"],\"side\":\"BOTTOM\"},\"type\":\"ConnectorPlacement.EquallySpacedRectSide\",\"uuid\":\"6d61618f-1cbe-4c91-8d9a-cf1c63ddd154\"}]},\"type\":\"ConnectorPlacement.EquallySpacedConnector\",\"uuid\":\"3aecd3e6-ec94-4a95-ad20-92352af1806b\"}],\"packageUris\":[\"http://schema.mathworks.com/mf0/Connector/R2020b\"],\"version\":\"1.0\"}"
  sensRL : Subsystem
      settings: PortSchema="{\"entries\":[{\"content\":{\"sides\":[{\"content\":{\"connectorIds\":[]},\"type\":\"ConnectorPlacement.EquallySpacedRectSide\",\"uuid\":\"bd83465d-2bef-45ec-b31a-ccd96dc04922\"},{\"content\":{\"connectorIds\":[],\"side\":\"RIGHT\"},\"type\":\"ConnectorPlacement.EquallySpacedRectSide\",\"uuid\":\"7d39c37e-7359-45a9-8850-f640f6442332\"},{\"content\":{\"connectorIds\":[\"LConn1\"],\"side\":\"TOP\"},\"type\":\"ConnectorPlacement.EquallySpacedRectSide\",\"uuid\":\"9171d6ae-b8cc-4ed2-b32d-fb0addba6640\"},{\"content\":{\"connectorIds\":[\"Out1\",\"RConn1\"],\"side\":\"BOTTOM\"},\"type\":\"ConnectorPlacement.EquallySpacedRectSide\",\"uuid\":\"6d61618f-1cbe-4c91-8d9a-cf1c63ddd154\"}]},\"type\":\"ConnectorPlacement.EquallySpacedConnector\",\"uuid\":\"3aecd3e6-ec94-4a95-ad20-92352af1806b\"}],\"packageUris\":[\"http://schema.mathworks.com/mf0/Connector/R2020b\"],\"version\":\"1.0\"}"
  sensRR : Subsystem
      settings: PortSchema="{\"entries\":[{\"content\":{\"sides\":[{\"content\":{\"connectorIds\":[]},\"type\":\"ConnectorPlacement.EquallySpacedRectSide\",\"uuid\":\"bd83465d-2bef-45ec-b31a-ccd96dc04922\"},{\"content\":{\"connectorIds\":[],\"side\":\"RIGHT\"},\"type\":\"ConnectorPlacement.EquallySpacedRectSide\",\"uuid\":\"7d39c37e-7359-45a9-8850-f640f6442332\"},{\"content\":{\"connectorIds\":[\"LConn1\"],\"side\":\"TOP\"},\"type\":\"ConnectorPlacement.EquallySpacedRectSide\",\"uuid\":\"9171d6ae-b8cc-4ed2-b32d-fb0addba6640\"},{\"content\":{\"connectorIds\":[\"Out1\",\"RConn1\"],\"side\":\"BOTTOM\"},\"type\":\"ConnectorPlacement.EquallySpacedRectSide\",\"uuid\":\"6d61618f-1cbe-4c91-8d9a-cf1c63ddd154\"}]},\"type\":\"ConnectorPlacement.EquallySpacedConnector\",\"uuid\":\"3aecd3e6-ec94-4a95-ad20-92352af1806b\"}],\"packageUris\":[\"http://schema.mathworks.com/mf0/Connector/R2020b\"],\"version\":\"1.0\"}"
  Center : PMIOPort  Side=Right
  feet : PMIOPort  Port=2  Side=Right
  footSens : Outport
  wires:
  [refFR] -> FR/1(In1)  "refFR"
  [refFL] -> FL/1(In1)  "refFL"
  [refRR] -> RR/1(In1)  "refRR"
  [refRL] -> RL/1(In1)  "refRL"
  Bus Creator/1 -> footSens/1
  FootFR/1(sensor) -> Bus Creator/2
  FootFL/1(sensor) -> Bus Creator/5
  FootRL/1(sensor) -> Bus Creator/8
  FootRR/1(sensor) -> Bus Creator/11
  sensFR/1(bend) -> Bus Creator/3
  sensFL/1(bend) -> Bus Creator/6
  sensRL/1(bend) -> Bus Creator/9
  sensRR/1(bend) -> Bus Creator/12
  Demux/1 -> [refFR]
  Demux/2 -> [refFL]
  Demux/3 -> [refRL]
  Demux/4 -> [refRR]
  motorRefs/1 -> Demux/1  "Refs"
  FR/1(powers) -> Bus Creator/1  "powerFR"
  FL/1(powers) -> Bus Creator/4  "powerFL"
  RL/1(powers) -> Bus Creator/7  "powerRL"
  RR/1(powers) -> Bus Creator/10  "powerRR"
  connections:
  sensFL/LConn1 -- FL/LConn1 -- Rigid Transform4/LConn1
  sensRR/LConn1 -- RR/LConn1 -- Rigid Transform3/LConn1
  sensRL/LConn1 -- RL/LConn1 -- Rigid Transform2/LConn1
  FootFR/LConn1 -- FootFL/LConn1 -- feet/RConn1 -- FootRR/LConn1 -- FootRL/LConn1
  sensFL/RConn1 -- FL/RConn1 -- FootFL/RConn1
  sensRL/RConn1 -- RL/RConn1 -- FootRL/RConn1
  sensRR/RConn1 -- RR/RConn1 -- FootRR/RConn1
  Rigid Transform2/RConn1 -- Rigid Transform3/RConn1 -- Rigid Transform1/LConn1 -- Rigid Transform5/RConn1 -- Rigid Transform4/RConn1
  Rigid Transform/LConn1 -- StructureDisk/LConn1
  StructureDisk/RConn1 -- Rigid Transform1/RConn1
  Rigid Transform/RConn1 -- 6-DOF Joint/RConn1 -- Center/RConn1
  FR/LConn1 -- sensFR/LConn1 -- Rigid Transform5/LConn1
  FR/RConn1 -- FootFR/RConn1 -- sensFR/RConn1
  Rigid Transform9/RConn1 -- 6-DOF Joint/LConn1
  Rigid Transform9/LConn1 -- World Frame/RConn1

== system RLvali_2021bold/Sensors1 ==
  LegSens : Inport
  Bus Creator1 : BusCreator  Inputs=8
  COT : Subsystem
  Derivative3 : Derivative
  Derivative4 : Derivative
  Derivative5 : Derivative
  Mux : Mux  Inputs=7
  PS-Simulink Converter{1,4..5,7} (4 alike) : nesl_utility/PS-Simulink Converter  PhysicalDomain=network_engine_domain  SubClassName=ps_output  LeftPortType=input  RightPortType=output  PseudoPeriodic=off  Frequencies=[]  Unit=1  AffineConversion=off
      settings: SourceProductBaseCode=PW,SS
  Rate Transition : RateTransition  OutPortSampleTime=Ts
  To Workspace1 : ToWorkspace  VariableName=Observations  SaveFormat=Timeseries  SampleTime=Ts
      settings: Save2DSignal=2-D array (concatenate along first dimension)
  Transform Sensor : sm_lib/Frames and Transforms/Transform Sensor  MeasurementFrame=World  SenseAngle=off  SenseAxis=off  SenseAngle1=off  SenseAngle2=off  SenseAngle3=off  SenseQ=on  SenseR=off  SenseOmegaX=off  SenseOmegaY=off  SenseOmegaZ=off  SenseOmega1=off  SenseOmega2=off  SenseOmega3=off  SenseQDot=off  SenseRDot=off  SenseAlphaX=off  SenseAlphaY=off  SenseAlphaZ=off  SenseAlpha1=off  SenseAlpha2=off  SenseAlpha3=off  SenseQDDot=off  SenseRDDot=off  SenseX=on  SenseY=on  SenseZ=on  SenseRad=off  SenseAzim=off  SenseDist=off  SenseInc=off  SenseXDot=off  SenseYDot=off  SenseZDot=off  SenseRadDot=off  SenseAzimDot=off  SenseDistDot=off  SenseIncDot=off  SenseXDDot=off  SenseYDDot=off  SenseZDDot=off  SenseRadDDot=off  SenseAzimDDot=off  SenseDistDDot=off  SenseIncDDot=off
  q2r : MATLAB Function  TreatAsAtomicUnit=on
  F : PMIOPort  Side=Left
  B : PMIOPort  Port=2  Side=Left
  sen : Outport  VectorParamsAs1DForOutWhenUnconnected=off
  tag scope: x_pos=global
  wires:
  PS-Simulink Converter1/1 -> q2r/1(u)  "q"
  PS-Simulink Converter5/1 -> Derivative5/1, Bus Creator1/4, Mux/4  "z"
  PS-Simulink Converter4/1 -> Bus Creator1/3, Mux/3, Derivative4/1  "y"
  PS-Simulink Converter7/1 -> [x_pos], Bus Creator1/2, Mux/2, Derivative3/1  "x"
  Bus Creator1/1 -> Rate Transition/1
  Rate Transition/1 -> sen/1
  Derivative3/1 -> Bus Creator1/5, Mux/5  "vx"
  Derivative4/1 -> Bus Creator1/6, Mux/6  "vy"
  Derivative5/1 -> Bus Creator1/7, Mux/7  "vz"
  LegSens/1 -> COT/1(SigsFromLegs), Bus Creator1/8  "SigsFromLegs"
  q2r/1(y) -> Bus Creator1/1, Mux/1  "rot"
  Mux/1 -> To Workspace1/1
  connections:
  F/RConn1 -- Transform Sensor/RConn1
  B/RConn1 -- Transform Sensor/LConn1
  PS-Simulink Converter1/LConn1 -- Transform Sensor/RConn2
  Transform Sensor/RConn3 -- PS-Simulink Converter7/LConn1
  PS-Simulink Converter4/LConn1 -- Transform Sensor/RConn4
  PS-Simulink Converter5/LConn1 -- Transform Sensor/RConn5

== system RLvali_2021bold/floor1 ==
  Grid Plane : Subsystem  Description=Grid block, GA, 2021  mask(Grid Block){length=floor_length, width=floor_width, numSqrs=2, lineWidth=0.005, gridColor=[0.6 0.6 0.6], gridOpacity=0.7, planeColor=[0.8 1.0 1.0], planeOpacity=1}
      mask prompts: length "Length (m)"; width "Width (m)"; numSqrs "Number of Squares"; lineWidth "Line Width (m)"; gridColor "Grid Color [R G B]"; gridOpacity "Grid Opacity"; planeColor "Plane Color [R G B]"; planeOpacity "Plane Opacity"
      mask help:
      | This block creates a grid plane using the Extr_Data_Mesh() function included in the "Simscape Multibody Parts Library" add-on. Please make sure that you have that add-on installed before using this block.
      | Georgios Andrikopoulos, KTH, 2021
      mask init:
      | box_h = (length - ...
      |     (lineWidth*(numSqrs+1)))/...
      |     numSqrs;
      | box_l = (length - ...
      |     (lineWidth*(1+1)))/1;
      | layer1 = Extr_Data_Mesh(width,...
      |     width,numSqrs,1,...
      |     box_h,box_l);
      | 
      | box_h2 = (length - ...
      |     ((lineWidth/3)*((numSqrs*10)+1)))/...
      |     (numSqrs*10);
      | box_l2 = (length - ...
      |     ((lineWidth/3)*(1+1)))/1;
      | layer2 = Extr_Data_Mesh(width,...
      |     width,(numSqrs*10),1,...
      |     box_h2,box_l2);
      | 
      | box_h3 = (length - ...
      |     ((lineWidth/20)*((numSqrs*100)+1)))/...
      |     (numSqrs*100);
      | box_l3 = (length - ...
      |     ((lineWidth/20)*(1+1)))/1;
      | layer3 = Extr_Data_Mesh(width,...
      |     width,(numSqrs*100),1,...
      |     box_h3,box_l3);
  worldSetting : Subsystem
  world : PMIOPort  Side=Left
  flor : PMIOPort  Port=2  Side=Right
  connections:
  Grid Plane/RConn1 -- flor/RConn1
  world/RConn1 -- Grid Plane/LConn1 -- worldSetting/RConn1

== system RLvali_2021bold/Act2Angle/DecideToUseExt ==
  Clock : Clock
  Constant : Constant  Value=isUseExtAct
  Constant1 : Constant  Value=0
  Constant2 : Constant
  Constant3 : Constant  Value=0
  Switch : Switch  Criteria=u2 > Threshold  Threshold=startAgentTime
  Switch1 : Switch  Criteria=u2 > Threshold
  Out1 : Outport
  wires:
  Constant/1 -> Switch1/2
  Switch1/1 -> Out1/1
  Constant2/1 -> Switch/3
  Constant1/1 -> Switch/1
  Clock/1 -> Switch/2
  Constant3/1 -> Switch1/3
  Switch/1 -> Switch1/1

== system RLvali_2021bold/Act2Angle/Human expert ==
  Mux10 : Mux
  alpha_b : simulink/Sources/Repeating Sequence  rep_seq_t=[0 0.2 0.4 0.6 0.8]  rep_seq_y=[0.5 1 0.5 0 0.5]
  alpha_b1 : simulink/Sources/Repeating Sequence  rep_seq_t=[0 0.2 0.4 0.6 0.8]  rep_seq_y=[0.5 0 0.5 1 0.5]
  z_l : simulink/Sources/Repeating Sequence  rep_seq_t=[0 0.2 0.4 0.6 0.8]  rep_seq_y=[0 1 1 1 0]
  z_l1 : simulink/Sources/Repeating Sequence  rep_seq_t=[0 0.2 0.4 0.6 0.8]  rep_seq_y=[1 1 0 1 1]
  Out1 : Outport
  wires:
  Mux10/1 -> Out1/1
  alpha_b/1 -> Mux10/1  "alpha_b_Ref"
  z_l1/1 -> Mux10/4  "z_l_Ref"
  z_l/1 -> Mux10/2  "z_l_Ref"
  alpha_b1/1 -> Mux10/3  "alpha_b_Ref"

== system RLvali_2021bold/Act2Angle/Human expert1 ==
  Mux2 : Mux
  Subsystem : Subsystem
  Subsystem1 : Subsystem  Commented=on
  alpha_b : simulink/Sources/Repeating Sequence  rep_seq_t=[0 0.2 0.4 0.6 0.8]  rep_seq_y=[0 1 0 -1 0]
  alpha_b1 : simulink/Sources/Repeating Sequence  rep_seq_t=[0 0.2 0.4 0.6 0.8]  rep_seq_y=[0 -1 0 1 0]
  z_l : simulink/Sources/Repeating Sequence  rep_seq_t=[0 0.2 0.4 0.6 0.8]  rep_seq_y=[-1 1 1 1 -1]
  z_l1 : simulink/Sources/Repeating Sequence  rep_seq_t=[0 0.2 0.4 0.6 0.8]  rep_seq_y=[1 1 -1 1 1]
  Inport : Outport
  wires:
  z_l1/1 -> Mux2/4  "z_l_Ref"
  z_l/1 -> Mux2/2  "z_l_Ref"
  Mux2/1 -> Subsystem/1(-1~1)
  alpha_b/1 -> Mux2/1  "alpha_b_Ref"
  alpha_b1/1 -> Mux2/3  "alpha_b_Ref"
  Subsystem/1(0~1) -> Inport/1

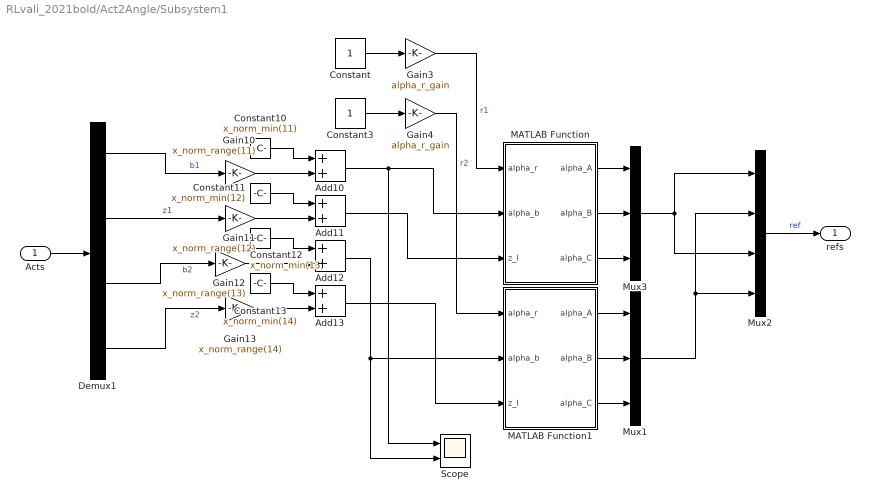
== system RLvali_2021bold/Act2Angle/Subsystem1 ==
  Acts : Inport
  Add{10..13} (4 alike) : Sum
  Constant : Constant
  Constant10 : Constant  Value=x_norm_min(11)
  Constant11 : Constant  Value=x_norm_min(12)
  Constant12 : Constant  Value=x_norm_min(13)
  Constant13 : Constant  Value=x_norm_min(14)
  Constant3 : Constant
  Demux1 : Demux
  Gain10 : Gain  Gain=x_norm_range(11)
  Gain11 : Gain  Gain=x_norm_range(12)
  Gain12 : Gain  Gain=x_norm_range(13)
  Gain13 : Gain  Gain=x_norm_range(14)
  Gain3 : Gain  Gain=alpha_r_gain
  Gain4 : Gain  Gain=alpha_r_gain
  MATLAB Function : MATLAB Function  TreatAsAtomicUnit=on
  MATLAB Function1 : MATLAB Function  TreatAsAtomicUnit=on
  Mux1 : Mux  Inputs=3
  Mux2 : Mux
  Mux3 : Mux  Inputs=3
  Scope : Scope  NumInputPorts=2
  refs : Outport
  wires:
  Acts/1 -> Demux1/1
  Mux2/1 -> refs/1  "ref"
  Gain4/1 -> MATLAB Function1/1(alpha_r)  "r2"
  MATLAB Function1/1(alpha_A) -> Mux1/1
  Gain3/1 -> MATLAB Function/1(alpha_r)  "r1"
  MATLAB Function/3(alpha_C) -> Mux3/3
  MATLAB Function1/3(alpha_C) -> Mux1/3
  MATLAB Function/1(alpha_A) -> Mux3/1
  MATLAB Function/2(alpha_B) -> Mux3/2
  MATLAB Function1/2(alpha_B) -> Mux1/2
  Mux3/1 -> Mux2/1, Mux2/3
  Mux1/1 -> Mux2/4, Mux2/2
  Constant/1 -> Gain3/1
  Constant3/1 -> Gain4/1
  Gain13/1 -> Add13/2
  Demux1/4 -> Gain13/1  "z2"
  Gain10/1 -> Add10/2
  Demux1/1 -> Gain10/1  "b1"
  Add11/1 -> MATLAB Function/3(z_l)
  Add13/1 -> MATLAB Function1/3(z_l)
  Gain12/1 -> Add12/2
  Demux1/2 -> Gain11/1  "z1"
  Demux1/3 -> Gain12/1  "b2"
  Gain11/1 -> Add11/2
  Constant10/1 -> Add10/1
  Constant12/1 -> Add12/1
  Constant11/1 -> Add11/1
  Constant13/1 -> Add13/1
  Add10/1 -> Scope/1, MATLAB Function/2(alpha_b)
  Add12/1 -> Scope/2, MATLAB Function1/2(alpha_b)

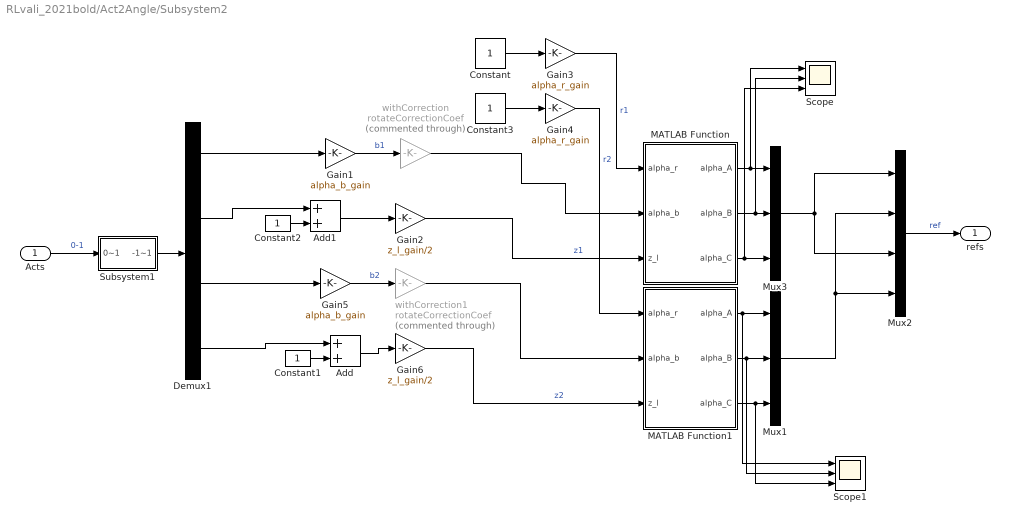
== system RLvali_2021bold/Act2Angle/Subsystem2 ==
  Acts : Inport
  Add : Sum
  Add1 : Sum
  Constant{,1..3} (4 alike) : Constant
  Demux1 : Demux
  Gain1 : Gain  Gain=alpha_b_gain
  Gain2 : Gain  Gain=z_l_gain/2
  Gain3 : Gain  Gain=alpha_r_gain
  Gain4 : Gain  Gain=alpha_r_gain
  Gain5 : Gain  Gain=alpha_b_gain
  Gain6 : Gain  Gain=z_l_gain/2
  MATLAB Function : MATLAB Function  TreatAsAtomicUnit=on
  MATLAB Function1 : MATLAB Function  TreatAsAtomicUnit=on
  Mux1 : Mux  Inputs=3
  Mux2 : Mux
  Mux3 : Mux  Inputs=3
  Scope : Scope  NumInputPorts=3
  Scope1 : Scope  NumInputPorts=3
  Subsystem1 : Subsystem
  withCorrection : Gain  Commented=through  Gain=rotateCorrectionCoef
  withCorrection1 : Gain  Commented=through  Gain=rotateCorrectionCoef
  refs : Outport
  wires:
  Gain6/1 -> MATLAB Function1/3(z_l)  "z2"
  Mux2/1 -> refs/1  "ref"
  Gain2/1 -> MATLAB Function/3(z_l)  "z1"
  Gain4/1 -> MATLAB Function1/1(alpha_r)  "r2"
  Gain3/1 -> MATLAB Function/1(alpha_r)  "r1"
  Gain1/1 -> withCorrection/1  "b1"
  MATLAB Function/3(alpha_C) -> Mux3/3, Scope/3
  MATLAB Function1/3(alpha_C) -> Scope1/3, Mux1/3
  MATLAB Function/1(alpha_A) -> Scope/1, Mux3/1
  MATLAB Function/2(alpha_B) -> Scope/2, Mux3/2
  MATLAB Function1/2(alpha_B) -> Mux1/2, Scope1/2
  Mux3/1 -> Mux2/1, Mux2/3
  Mux1/1 -> Mux2/4, Mux2/2
  Constant/1 -> Gain3/1
  Constant3/1 -> Gain4/1
  Gain5/1 -> withCorrection1/1  "b2"
  withCorrection/1 -> MATLAB Function/2(alpha_b)
  withCorrection1/1 -> MATLAB Function1/2(alpha_b)
  Acts/1 -> Subsystem1/1(0~1)  "0-1"
  Demux1/1 -> Gain1/1
  Demux1/3 -> Gain5/1
  Demux1/4 -> Add/1
  Constant1/1 -> Add/2
  Add/1 -> Gain6/1
  Demux1/2 -> Add1/1
  Constant2/1 -> Add1/2
  Add1/1 -> Gain2/1
  MATLAB Function1/1(alpha_A) -> Mux1/1, Scope1/1
  Subsystem1/1(-1~1) -> Demux1/1

== system RLvali_2021bold/Act2Angle/action2angle ==
  In1 : Inport
  Add : Sum  Inputs=+-
  Constant2 : Constant  Value=0.5
  withCorrection : Gain  Gain=angle_amp/0.5*rotateCorrectionCoef
  currAct_vec : Outport
  wires:
  In1/1 -> Add/1
  Constant2/1 -> Add/2
  Add/1 -> withCorrection/1
  withCorrection/1 -> currAct_vec/1
